simulink model "simulacion"  (R2017a)
settings: Solver=ode45  StartTime=0.0  StopTime=10.0  RelTol=1e-3  EnableMultiTasking=on
libraries: fl_lib x11, nesl_utility x6
settings Model: Creator=sala3  LastModifiedBy=Jesus
settings DataIOCC: LimitDataPoints=on  SaveFormat=Array
settings OptimizationCC: LifeSpan=inf
settings DebuggingCC: SFUnexpectedBacktrackingDiag=warning  SFNoUnconditionalDefaultTransitionDiag=warning  SFExecutionAtInitializationDiag=none
settings HardwareCC: ProdBitPerPointer=32  ProdBitPerSizeT=32  ProdBitPerPtrDiffT=32  ProdLargestAtomicFloat=None  ProdIntDivRoundTo=Undefined  ProdEndianess=Unspecified  ProdWordSize=32  ProdHWDeviceType=32-bit Generic
settings ModelReferenceCC: PropagateSignalLabelsOutOfModel=off
settings GRTTargetCC: TargetLangStandard=C89/C90 (ANSI)  GeneratePreprocessorConditionals=Disable all
settings ConfigComp: CovMetricSettings=dw  CovHtmlReporting=on  CovSaveCumulativeToWorkspaceVar=on  CovSaveSingleToWorkspaceVar=on  CovExternalEMLEnable=off

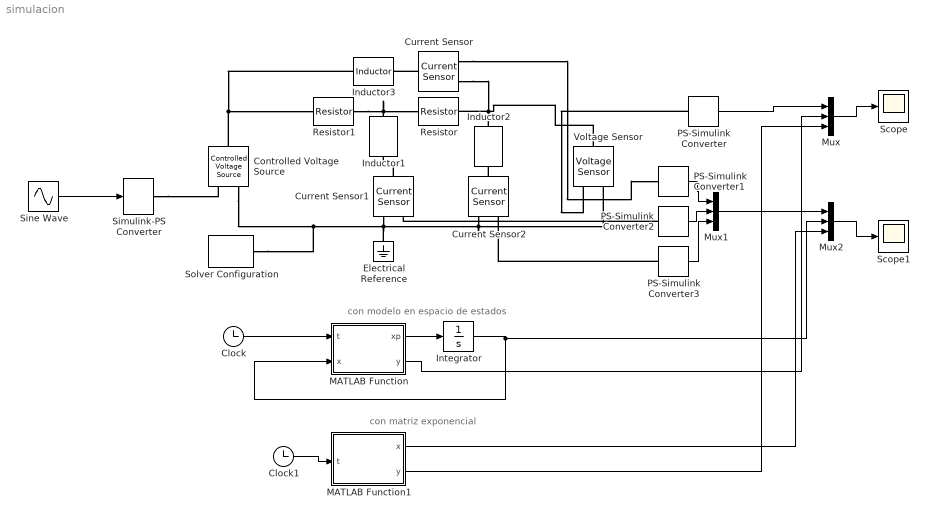
== system simulacion ==
  note: con modelo en espacio de estados
  note: con matriz exponencial
  Clock : Clock
  Clock1 : Clock
  Controlled Voltage Source : fl_lib/Electrical/Electrical Sources/Controlled Voltage Source
  Current Sensor : fl_lib/Electrical/Electrical Sensors/Current Sensor
  Current Sensor1 : fl_lib/Electrical/Electrical Sensors/Current Sensor
  Current Sensor2 : fl_lib/Electrical/Electrical Sensors/Current Sensor
  Electrical Reference : fl_lib/Electrical/Electrical Elements/Electrical Reference
  Inductor1 : fl_lib/Electrical/Electrical Elements/Inductor  l=1 H  r=0 Ohm  g=1e-9 1/Ohm  i_specify=off  i_priority=None  i=1 A  i_nominal_specify=off  i_nominal_unit=A  i_nominal_value=1  v_specify=off  v_priority=None  v=0 V  v_nominal_specify=off  v_nominal_unit=V  v_nominal_value=1  i_L_specify=on  i_L_priority=High  i_L=1 A  i_L_nominal_specify=off  i_L_nominal_unit=A  i_L_nominal_value=1
  Inductor2 : fl_lib/Electrical/Electrical Elements/Inductor  l=1 H  r=0 Ohm  g=1e-9 1/Ohm  i_specify=off  i_priority=None  i=1 A  i_nominal_specify=off  i_nominal_unit=A  i_nominal_value=1  v_specify=off  v_priority=None  v=0 V  v_nominal_specify=off  v_nominal_unit=V  v_nominal_value=1  i_L_specify=on  i_L_priority=High  i_L=1 A  i_L_nominal_specify=off  i_L_nominal_unit=A  i_L_nominal_value=1
  Inductor3 : fl_lib/Electrical/Electrical Elements/Inductor  l=1 H  r=0 Ohm  g=1e-9 1/Ohm  i_specify=off  i_priority=None  i=1 A  i_nominal_specify=off  i_nominal_unit=A  i_nominal_value=1  v_specify=off  v_priority=None  v=0 V  v_nominal_specify=off  v_nominal_unit=V  v_nominal_value=1  i_L_specify=on  i_L_priority=High  i_L=1 A  i_L_nominal_specify=off  i_L_nominal_unit=A  i_L_nominal_value=1
  Integrator : Integrator  InitialCondition=[1 1 1]
  MATLAB Function : MATLAB Function  TreatAsAtomicUnit=on
  MATLAB Function1 : MATLAB Function  TreatAsAtomicUnit=on
  Mux : Mux  Inputs=3
  Mux1 : Mux  Inputs=3
  Mux2 : Mux  Inputs=3
  PS-Simulink Converter{,1..3} (4 alike) : nesl_utility/PS-Simulink Converter  PhysicalDomain=network_engine_domain  SubClassName=ps_output  LeftPortType=input  RightPortType=output  PseudoPeriodic=off  Frequencies=[]  Unit=1  AffineConversion=off
  Resistor : fl_lib/Electrical/Electrical Elements/Resistor  R=1 Ohm  i_specify=off  i_priority=High  i=0 A  i_nominal_specify=off  i_nominal_unit=A  i_nominal_value=1  v_specify=off  v_priority=High  v=0 V  v_nominal_specify=off  v_nominal_unit=V  v_nominal_value=1
  Resistor1 : fl_lib/Electrical/Electrical Elements/Resistor  R=1 Ohm  i_specify=off  i_priority=High  i=0 A  i_nominal_specify=off  i_nominal_unit=A  i_nominal_value=1  v_specify=off  v_priority=High  v=0 V  v_nominal_specify=off  v_nominal_unit=V  v_nominal_value=1
  Scope : Scope
  Scope1 : Scope
  Simulink-PS Converter : nesl_utility/Simulink-PS Converter  PhysicalDomain=network_engine_domain  SubClassName=ps_input  LeftPortType=input  RightPortType=output  PseudoPeriodic=off  Frequencies=[]  NoiseDistribution=none  NoiseParameters=[]  Unit=1  AffineConversion=off  FilteringAndDerivatives=zero  SimscapeFilterOrder=1  InputFilterTimeConstant=0.001  UdotUserProvided=1
  Sine Wave : Sin  Amplitude=10  SampleTime=0
  Solver Configuration : nesl_utility/Solver Configuration  PhysicalDomain=network_engine_domain  SubClassName=solver  LeftPortType=input  RightPortType=generic  Accelerate=off  Tones=[]  Harmonics=[]  SimulateNoise=off  Profile=off  UseLocalSampling=off  EnableSwitchedLinearOptims=on  FrequencyDomain=off  UseCCode=off  RelTol=0.001  AbsTol=1e-06  MinStep=1e-09  ToWorkspace=off  RevertToSquareIcSolve=off  NumHomotopyIterations=100  PhasorMode=off  PhasorModeNumHarmonics=1  OverrideAbsTol=off  DoDC=off  ResidualTolerance=1e-09  UseLocalSolver=off  LocalSolverChoice=NE_BACKWARD_EULER_ADVANCER  LocalSolverSampleTime=0.001  DoFixedCost=off  MaxNonlinIter=3  MaxModeIter=2  LinearAlgebra=Sparse  DelaysMemoryBudget=1024  AutomaticFiltering=on  FilteringTimeConstant=0.001
  Voltage Sensor : fl_lib/Electrical/Electrical Sensors/Voltage Sensor
  wires:
  Sine Wave/1 -> Simulink-PS Converter/1
  Integrator/1 -> Mux2/2, MATLAB Function/2(x)
  MATLAB Function/1(xp) -> Integrator/1
  Clock/1 -> MATLAB Function/1(t)
  Mux/1 -> Scope/1
  PS-Simulink Converter/1 -> Mux/1
  MATLAB Function/2(y) -> Mux/2
  PS-Simulink Converter1/1 -> Mux1/1
  PS-Simulink Converter2/1 -> Mux1/2
  PS-Simulink Converter3/1 -> Mux1/3
  Mux1/1 -> Mux2/1
  Mux2/1 -> Scope1/1
  Clock1/1 -> MATLAB Function1/1(t)
  MATLAB Function1/1(x) -> Mux2/3
  MATLAB Function1/2(y) -> Mux/3
  connections:
  Voltage Sensor/LConn1 -- Inductor2/LConn1 -- Current Sensor/RConn2 -- Resistor/RConn1
  Inductor1/LConn1 -- Resistor/LConn1 -- Resistor1/RConn1
  Controlled Voltage Source/LConn1 -- Inductor3/LConn1 -- Resistor1/LConn1
  Controlled Voltage Source/RConn2 -- Current Sensor1/RConn2 -- Current Sensor2/RConn2 -- Voltage Sensor/RConn2 -- Electrical Reference/LConn1 -- Solver Configuration/RConn1
  PS-Simulink Converter/LConn1 -- Voltage Sensor/RConn1
  Simulink-PS Converter/RConn1 -- Controlled Voltage Source/RConn1
  Current Sensor/LConn1 -- Inductor3/RConn1
  Current Sensor1/LConn1 -- Inductor1/RConn1
  Current Sensor2/LConn1 -- Inductor2/RConn1
  Current Sensor/RConn1 -- PS-Simulink Converter1/LConn1
  PS-Simulink Converter2/LConn1 -- Current Sensor1/RConn1
  PS-Simulink Converter3/LConn1 -- Current Sensor2/RConn1

== matlab function simulacion/MATLAB Function1 ==
  data: x output; t input; y output
function [x,y]  = fcn(t)
%#codegen
x=real([(15*exp(-(5*t)/2)*cosh((17^(1/2)*t)/2))/13 - (10*sin(t))/13 - (80*cos(t))/13 + (121*17^(1/2)*exp(-(5*t)/2)*sinh((17^(1/2)*t)/2))/221 + 6;
 (40*sin(t))/13 - (70*cos(t))/13 + (70*exp(-(5*t)/2)*cosh((17^(1/2)*t)/2))/13 + exp(-(5*t)/2)*(cosh((17^(1/2)*t)/2) + (3*17^(1/2)*sinh((17^(1/2)*t)/2))/17) + (270*17^(1/2)*exp(-(5*t)/2)*sinh((17^(1/2)*t)/2))/221;
                                                                           (10*sin(t))/13 - (50*cos(t))/13 - (15*exp(-(5*t)/2)*cosh((17^(1/2)*t)/2))/13 - (121*17^(1/2)*exp(-(5*t)/2)*sinh((17^(1/2)*t)/2))/221 + 6]);
 y=(10*cos(t))/13 + (50*sin(t))/13 - (23*exp(-(5*t)/2)*cosh((17^(1/2)*t)/2))/13 + (175*17^(1/2)*exp(-(5*t)/2)*sinh((17^(1/2)*t)/2))/221;

== matlab function simulacion/MATLAB Function ==
  data: xp output; t input; y output; x input
function [xp,y] = fcn(t,x)
%#codegen
u=10*sin(t);
A=[-2 1 2;1 -1 -1;2 -1 -2]; 
B=[0 1 1]';
C=[0 0 1];
xp=A*x+B*u;
y=C*xp;
